simulink model "barra1Validation"  (R2018a)
settings: Solver=ode45  StartTime=0.0  StopTime=10  RelTol=1e-6  EnableMultiTasking=on
InitFcn:
  | barrassmodel= load('/Users/leonardopedroso/Desktop/CComp/Lab/1_identification/model/barrassmodel.mat');
  | nA3 = load('/Users/leonardopedroso/Desktop/CComp/Lab/1_identification/DATA/4_PlantModelIdentification18/identification.mat');
  | nA4 = load('/Users/leonardopedroso/Desktop/CComp/Lab/1_identification/DATA/4_PlantModelIdentification16/identification.mat');
settings Model: Creator=jomle  LastModifiedBy=leonardopedroso
settings DataIOCC: LimitDataPoints=on  SaveFormat=Array
settings OptimizationCC: LifeSpan=inf
settings DebuggingCC: SFUnexpectedBacktrackingDiag=warning  SFNoUnconditionalDefaultTransitionDiag=warning  SFExecutionAtInitializationDiag=none
settings HardwareCC: ProdBitPerPointer=32  ProdBitPerSizeT=32  ProdBitPerPtrDiffT=32  ProdLargestAtomicFloat=None  ProdIntDivRoundTo=Undefined  ProdEndianess=Unspecified  ProdWordSize=32  ProdHWDeviceType=32-bit Generic
settings ModelReferenceCC: PropagateSignalLabelsOutOfModel=off
settings CodeAppCC: StateflowObjectComments=on
settings GRTTargetCC: TargetLangStandard=C89/C90 (ANSI)  GeneratePreprocessorConditionals=Disable all
settings ConfigComp: CovMetricSettings=dw  CovHtmlReporting=on  CovSaveCumulativeToWorkspaceVar=on  CovSaveSingleToWorkspaceVar=on  CovExternalEMLEnable=off

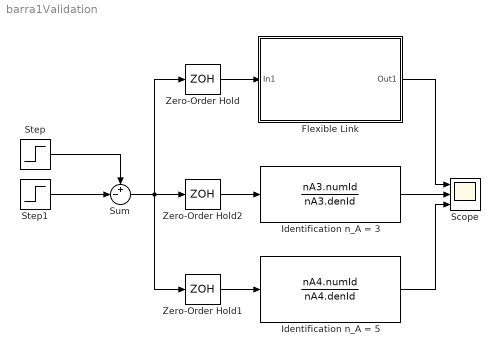
== system barra1Validation ==
  Flexible Link : Subsystem
      mask Display: image('./model/quanserlink.jpg');
  Identification n_A = 3 : DiscreteTransferFcn  Numerator=nA3.numId  Denominator=nA3.denId  SampleTime=0.02
  "Identification n_A = 5 " : DiscreteTransferFcn  Numerator=nA4.numId  Denominator=nA4.denId  SampleTime=0.01
  Scope : Scope  NumInputPorts=3
  Step : Step  SampleTime=0
  Step1 : Step  Time=1.5  SampleTime=0
  Sum : Sum  Inputs=+-|
  Zero-Order Hold : ZeroOrderHold  SampleTime=0.01
  Zero-Order Hold1 : ZeroOrderHold  SampleTime=0.01
  Zero-Order Hold2 : ZeroOrderHold  SampleTime=0.02
  wires:
  Flexible Link/1(Out1) -> Scope/1
  "Identification n_A = 5 "/1 -> Scope/3
  Zero-Order Hold/1 -> Flexible Link/1(In1)
  Zero-Order Hold2/1 -> Identification n_A = 3/1
  Zero-Order Hold1/1 -> "Identification n_A = 5 "/1
  Identification n_A = 3/1 -> Scope/2
  Step/1 -> Sum/1
  Step1/1 -> Sum/2
  Sum/1 -> Zero-Order Hold1/1, Zero-Order Hold/1, Zero-Order Hold2/1

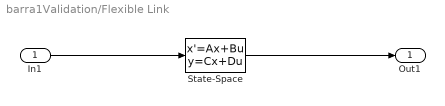
== system barra1Validation/Flexible Link ==
  In1 : Inport
  State-Space : StateSpace  A=barrassmodel.Atrue  B=barrassmodel.Btrue  C=barrassmodel.Ctrue  D=barrassmodel.Dtrue  InitialCondition=0
  Out1 : Outport
  wires:
  State-Space/1 -> Out1/1
  In1/1 -> State-Space/1
